simulink model "model_testslx_2015a"  (R2022a)
settings: Solver=ode3  StartTime=0.0  StopTime=100.0  FixedStep=0.01  RelTol=1e-3
values from neighbouring files (symbols this model uses):
  beta = params(1)    [model.m]
  g = 9.8105    [model.m]    (also in weryfikacja.m)
  I = 0.0226    [model.m]    (also in weryfikacja.m = 0.029572173408)
  K = params(3)    [model.m]
  tau = params(4)    [model.m]
  U = params(2)    [model.m]
settings Model: Creator=turgo  LastModifiedBy=turgo
settings SolverCC: AlgebraicLoopSolver=TrustRegion
settings OptimizationCC: LifeSpan=inf
settings DebuggingCC: SFExecutionAtInitializationDiag=none  SFMachineParentedDataDiag=warning  ArithmeticOperatorsInVariantConditions=warning
settings HardwareCC: ProdBitPerSizeT=32  ProdBitPerPtrDiffT=32  ProdWordSize=32  ProdHWDeviceType=Specified
settings SFSimCC: CustomCodeUndefinedFunction=UseInterfaceOnly
settings CodeAppCC: StateflowObjectComments=on

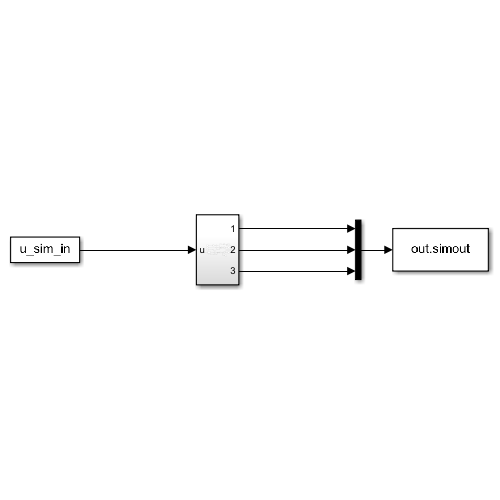
[thumbnail: Simulink's stored preview of the top-level diagram]
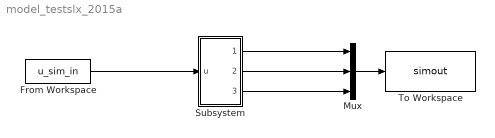
== system model_testslx_2015a ==
  From Workspace : FromWorkspace  VariableName=u_sim_in
  Mux : Mux  Inputs=3
  Subsystem : Subsystem
  To Workspace : ToWorkspace  VariableName=simout  SaveFormat=Structure With Time  SampleTime=-1
  wires:
  Mux/1 -> To Workspace/1
  Subsystem/1(Out1) -> Mux/1
  Subsystem/2(Out2) -> Mux/2
  Subsystem/3(Out3) -> Mux/3
  From Workspace/1 -> Subsystem/1(u)

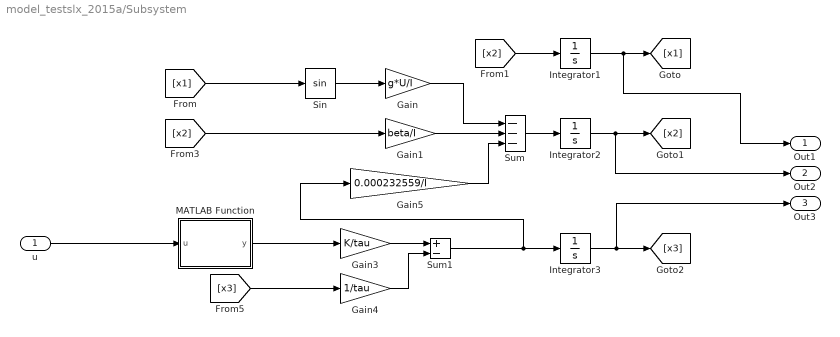
== system model_testslx_2015a/Subsystem ==
  u : Inport
  Gain : Gain  Gain=g*U/I
  Gain1 : Gain  Gain=beta/I
  Gain3 : Gain  Gain=K/tau
  Gain4 : Gain  Gain=1/tau
  Gain5 : Gain  Gain=0.000232559/I
  Integrator1 : Integrator
  Integrator2 : Integrator
  Integrator3 : Integrator
  MATLAB Function : MATLAB Function  TreatAsAtomicUnit=on
  Sin : Trigonometry
  Sum : Sum  Inputs=---
  Sum1 : Sum  Inputs=+-
  Out1 : Outport
  Out2 : Outport  Port=2
  Out3 : Outport  Port=3
  wires:
  [x1] -> Sin/1
  Integrator1/1 -> Out1/1, [x1]
  Sum/1 -> Integrator2/1
  Sin/1 -> Gain/1
  Gain/1 -> Sum/1
  Gain5/1 -> Sum/3
  Gain4/1 -> Sum1/2
  Gain3/1 -> Sum1/1
  [x2] -> Gain1/1
  [x2] -> Integrator1/1
  Integrator3/1 -> Out3/1, [x3]
  Gain1/1 -> Sum/2
  Integrator2/1 -> Out2/1, [x2]
  u/1 -> MATLAB Function/1(u)
  Sum1/1 -> Gain5/1, Integrator3/1
  MATLAB Function/1(y) -> Gain3/1
  [x3] -> Gain4/1

== matlab function model_testslx_2015a/Subsystem/MATLAB Function ==
  data: u input; y output
function y = fcn(u)

y = 211.6*u + 0.953;
